simulink model "Closed_loop_PI"  (R2020b)
settings: Solver=VariableStepAuto  StartTime=0.0  StopTime=10.0  RelTol=1e-3
model workspace (MAT data in the model file):
  A = 1
  Ap = 1.0472
  T = 2
  Th = 1
  Ti = 2
libraries: cstblocks x1
settings Model: Creator=kocka  LastModifiedBy=kocka

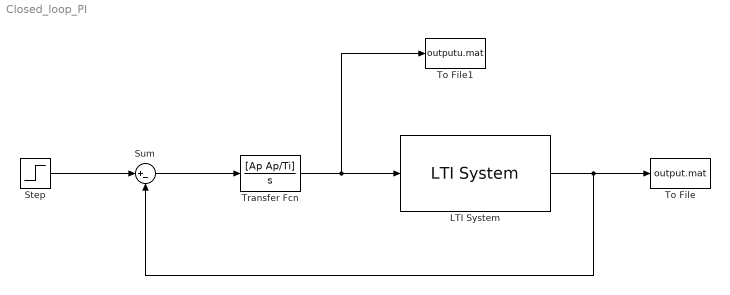
== system Closed_loop_PI ==
  LTI System : cstblocks/LTI System  sys="tf(A, [T 1], \"iodelay\", Th)"  IC=[]
  Step : Step  Time=0  SampleTime=0
  Sum : Sum  Inputs=|+-
  To File : ToFile  Filename=output.mat  MatrixName=y
  To File1 : ToFile  Filename=outputu.mat  MatrixName=u
  Transfer Fcn : TransferFcn  Numerator=[Ap Ap/Ti]  Denominator=[1 0]
  wires:
  Step/1 -> Sum/1
  Sum/1 -> Transfer Fcn/1
  Transfer Fcn/1 -> To File1/1, LTI System/1
  LTI System/1 -> Sum/2, To File/1
